simulink model "Learning_Rate"  (R2021b)
settings: Solver=FixedStepAuto  StartTime=0.0  StopTime=1190  FixedStep=0.01  RelTol=1e-3
libraries: drivingcycle_lib x3
settings Model: Creator=Alireza  LastModifiedBy=Alireza

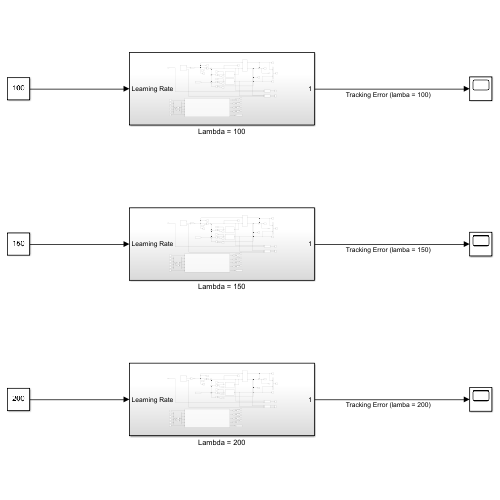
[thumbnail: Simulink's stored preview of the top-level diagram]
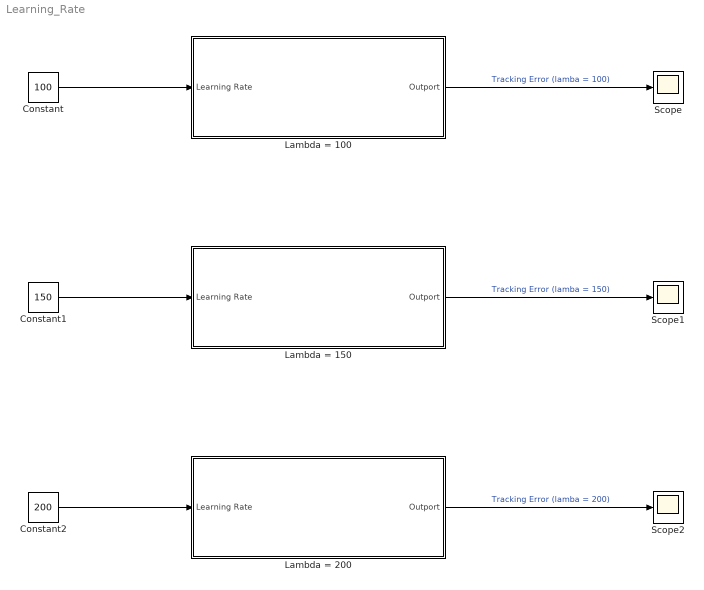
== system Learning_Rate ==
  Constant : Constant  Value=100
  Constant1 : Constant  Value=150
  Constant2 : Constant  Value=200
  Lambda = 100 : Subsystem
  Lambda = 150 : Subsystem
  Lambda = 200 : Subsystem
  Scope : Scope
  Scope1 : Scope
  Scope2 : Scope
  wires:
  Constant/1 -> Lambda = 100/1(Learning Rate)
  Constant1/1 -> Lambda = 150/1(Learning Rate)
  Constant2/1 -> Lambda = 200/1(Learning Rate)
  Lambda = 100/1(Outport) -> Scope/1  "Tracking Error (lamba = 100)"
  Lambda = 150/1(Outport) -> Scope1/1  "Tracking Error (lamba = 150)"
  Lambda = 200/1(Outport) -> Scope2/1  "Tracking Error (lamba = 200)"

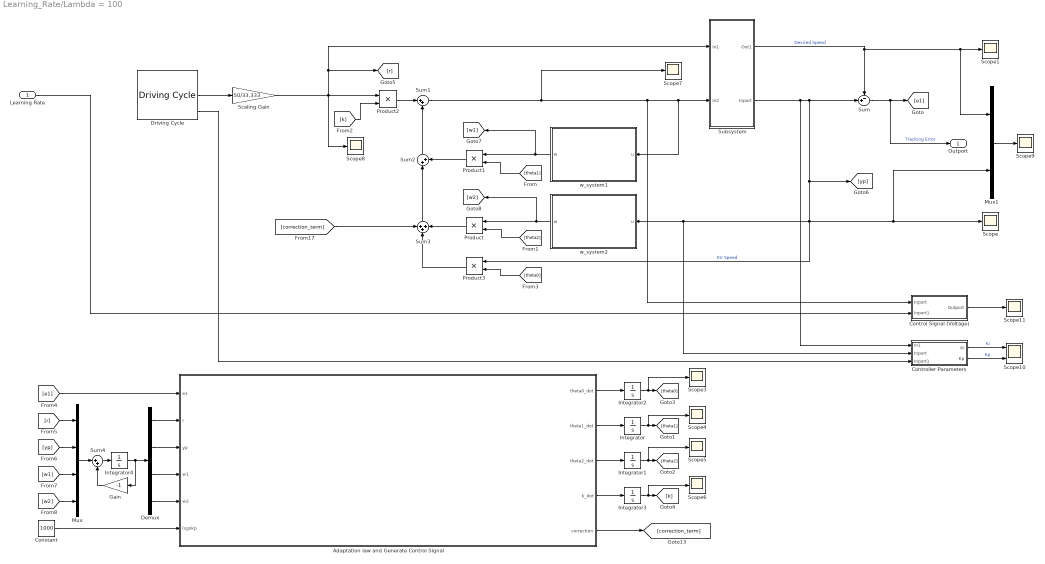
== system Learning_Rate/Lambda = 100 ==
  Learning Rate : Inport
  Adaptation law and Generate Control Signal : MATLAB Function  TreatAsAtomicUnit=on
  Constant : Constant  Value=1000
  Control Signal (Voltage) : Subsystem
  Controller Parameters : Subsystem
  Demux : Demux
  Driving Cycle : drivingcycle_lib/Driving Cycle  CycleName=NEDC  CycleRepeatsForever=off
      settings: SourceProductName=Driving Cycle Blockset
  Gain : Gain  Gain=-1
  Integrator{,1..4} (5 alike) : Integrator
  Mux : Mux
  Mux1 : Mux  Inputs=2
  Product{,1..3} (4 alike) : Product
  Scaling Gain : Gain  Gain=50/33.333
  Scope{,1,3..9,11} (10 alike) : Scope
  Scope10 : Scope  NumInputPorts=2
  Subsystem : Subsystem
  Sum : Sum  Inputs=-+|
  Sum1 : Sum  Inputs=|++
  Sum2 : Sum  Inputs=|++
  Sum3 : Sum  Inputs=+++
  Sum4 : Sum  Inputs=|++
  w_system1 : Subsystem  mask{lambda=-1, l=1}
      mask DialogControl lambda_name Prompt: Lambda:
      mask DialogControl l_name Prompt: L:
  w_system2 : Subsystem  mask{lambda=-1, l=1}
      mask DialogControl lambda_name Prompt: Lambda:
      mask DialogControl l_name Prompt: L:
  Outport : Outport
  wires:
  Subsystem/2(Inport) -> Controller Parameters/1(In1), Controller Parameters/2(Inport), w_system2/1(u), Product3/1, Mux1/2, Scope/1, [yp], Sum/2  "EV Speed"
  [w2] -> Mux/4
  Controller Parameters/2(Kp) -> Scope10/2  "Kp"
  Mux/1 -> Sum4/1
  Control Signal (Voltage)/1(Outport) -> Scope11/1
  Driving Cycle/2 -> Scaling Gain/1
  [e1] -> Adaptation law and Generate Control Signal/1(e1)
  Adaptation law and Generate Control Signal/1(theta0_dot) -> Integrator2/1
  Product/1 -> Sum3/3
  Integrator4/1 -> Gain/1, Demux/1
  Driving Cycle/3 -> Controller Parameters/3(Inport1)
  Controller Parameters/1(Ki) -> Scope10/1  "Ki"
  [correction_term] -> Sum3/1
  Gain/1 -> Sum4/2
  Sum1/1 -> Scope7/1, Control Signal (Voltage)/1(Inport), w_system1/1(u), Subsystem/2(In2)
  Adaptation law and Generate Control Signal/3(theta2_dot) -> Integrator1/1
  Product2/1 -> Sum1/1
  Integrator/1 -> Scope4/1, [theta1]
  w_system1/1(w) -> [w1], Product1/1
  Demux/3 -> Adaptation law and Generate Control Signal/4(w1)
  [r] -> Mux/1
  Product3/1 -> Sum3/2
  Demux/1 -> Adaptation law and Generate Control Signal/2(r)
  w_system2/1(w) -> [w2], Product/1
  Sum4/1 -> Integrator4/1
  Sum/1 -> Outport/1, [e1]  "Tracking Error"
  Subsystem/1(Out1) -> Sum/1, Mux1/1, Scope1/1  "Desired Speed"
  [theta0] -> Product3/2
  Sum2/1 -> Sum1/2
  Adaptation law and Generate Control Signal/4(k_dot) -> Integrator3/1
  [yp] -> Mux/2
  Demux/2 -> Adaptation law and Generate Control Signal/3(yp)
  Sum3/1 -> Sum2/1
  [k] -> Product2/2
  Adaptation law and Generate Control Signal/2(theta1_dot) -> Integrator/1
  Integrator3/1 -> Scope6/1, [k]
  [theta2] -> Product/2
  Mux1/1 -> Scope9/1
  Product1/1 -> Sum2/2
  [w1] -> Mux/3
  [theta1] -> Product1/2
  Adaptation law and Generate Control Signal/5(correction) -> [correction_term]
  Demux/4 -> Adaptation law and Generate Control Signal/5(w2)
  Integrator1/1 -> [theta2], Scope5/1
  Scaling Gain/1 -> Scope8/1, Subsystem/1(In1), [r], Product2/1
  Integrator2/1 -> [theta0], Scope3/1
  Constant/1 -> Adaptation law and Generate Control Signal/6(lsgnkp)
  Learning Rate/1 -> Control Signal (Voltage)/2(Inport1)

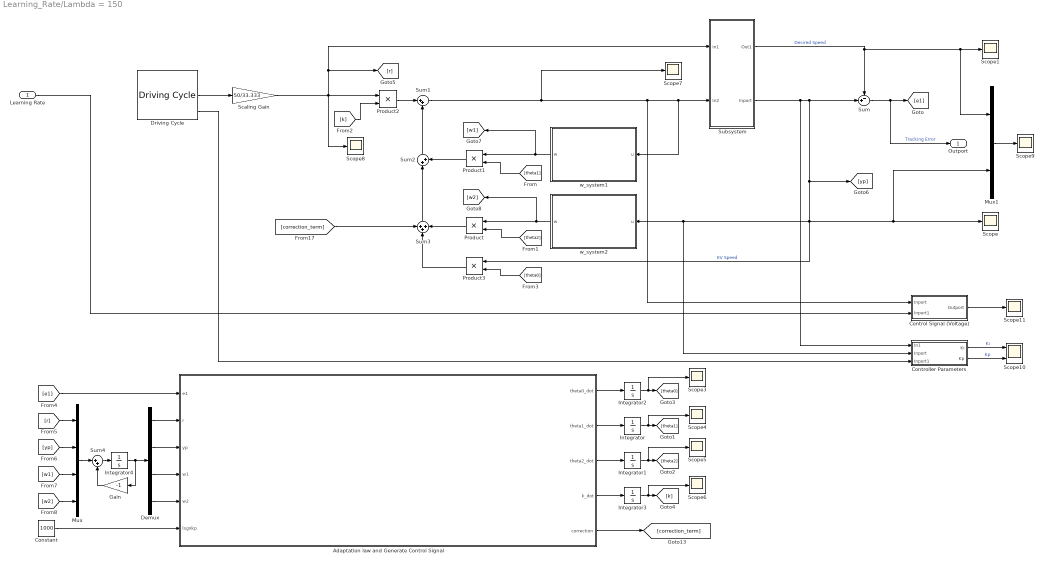
== system Learning_Rate/Lambda = 150 ==
  Learning Rate : Inport
  Adaptation law and Generate Control Signal : MATLAB Function  TreatAsAtomicUnit=on
  Constant : Constant  Value=1000
  Control Signal (Voltage) : Subsystem
  Controller Parameters : Subsystem
  Demux : Demux
  Driving Cycle : drivingcycle_lib/Driving Cycle  CycleName=NEDC  CycleRepeatsForever=off
      settings: SourceProductName=Driving Cycle Blockset
  Gain : Gain  Gain=-1
  Integrator{,1..4} (5 alike) : Integrator
  Mux : Mux
  Mux1 : Mux  Inputs=2
  Product{,1..3} (4 alike) : Product
  Scaling Gain : Gain  Gain=50/33.333
  Scope{,1,3..9,11} (10 alike) : Scope
  Scope10 : Scope  NumInputPorts=2
  Subsystem : Subsystem
  Sum : Sum  Inputs=-+|
  Sum1 : Sum  Inputs=|++
  Sum2 : Sum  Inputs=|++
  Sum3 : Sum  Inputs=+++
  Sum4 : Sum  Inputs=|++
  w_system1 : Subsystem  mask{lambda=-1, l=1}
      mask DialogControl lambda_name Prompt: Lambda:
      mask DialogControl l_name Prompt: L:
  w_system2 : Subsystem  mask{lambda=-1, l=1}
      mask DialogControl lambda_name Prompt: Lambda:
      mask DialogControl l_name Prompt: L:
  Outport : Outport
  wires:
  Subsystem/2(Inport) -> Controller Parameters/1(In1), Controller Parameters/2(Inport), w_system2/1(u), Product3/1, Mux1/2, Scope/1, [yp], Sum/2  "EV Speed"
  [w2] -> Mux/4
  Controller Parameters/2(Kp) -> Scope10/2  "Kp"
  Mux/1 -> Sum4/1
  Control Signal (Voltage)/1(Outport) -> Scope11/1
  Driving Cycle/2 -> Scaling Gain/1
  [e1] -> Adaptation law and Generate Control Signal/1(e1)
  Adaptation law and Generate Control Signal/1(theta0_dot) -> Integrator2/1
  Product/1 -> Sum3/3
  Integrator4/1 -> Gain/1, Demux/1
  Driving Cycle/3 -> Controller Parameters/3(Inport1)
  Controller Parameters/1(Ki) -> Scope10/1  "Ki"
  [correction_term] -> Sum3/1
  Gain/1 -> Sum4/2
  Sum1/1 -> Scope7/1, Control Signal (Voltage)/1(Inport), w_system1/1(u), Subsystem/2(In2)
  Adaptation law and Generate Control Signal/3(theta2_dot) -> Integrator1/1
  Product2/1 -> Sum1/1
  Integrator/1 -> Scope4/1, [theta1]
  w_system1/1(w) -> [w1], Product1/1
  Demux/3 -> Adaptation law and Generate Control Signal/4(w1)
  [r] -> Mux/1
  Product3/1 -> Sum3/2
  Demux/1 -> Adaptation law and Generate Control Signal/2(r)
  w_system2/1(w) -> [w2], Product/1
  Sum4/1 -> Integrator4/1
  Sum/1 -> Outport/1, [e1]  "Tracking Error"
  Subsystem/1(Out1) -> Sum/1, Mux1/1, Scope1/1  "Desired Speed"
  [theta0] -> Product3/2
  Sum2/1 -> Sum1/2
  Adaptation law and Generate Control Signal/4(k_dot) -> Integrator3/1
  [yp] -> Mux/2
  Demux/2 -> Adaptation law and Generate Control Signal/3(yp)
  Sum3/1 -> Sum2/1
  [k] -> Product2/2
  Adaptation law and Generate Control Signal/2(theta1_dot) -> Integrator/1
  Integrator3/1 -> Scope6/1, [k]
  [theta2] -> Product/2
  Mux1/1 -> Scope9/1
  Product1/1 -> Sum2/2
  [w1] -> Mux/3
  [theta1] -> Product1/2
  Adaptation law and Generate Control Signal/5(correction) -> [correction_term]
  Demux/4 -> Adaptation law and Generate Control Signal/5(w2)
  Integrator1/1 -> [theta2], Scope5/1
  Scaling Gain/1 -> Scope8/1, Subsystem/1(In1), [r], Product2/1
  Integrator2/1 -> [theta0], Scope3/1
  Constant/1 -> Adaptation law and Generate Control Signal/6(lsgnkp)
  Learning Rate/1 -> Control Signal (Voltage)/2(Inport1)

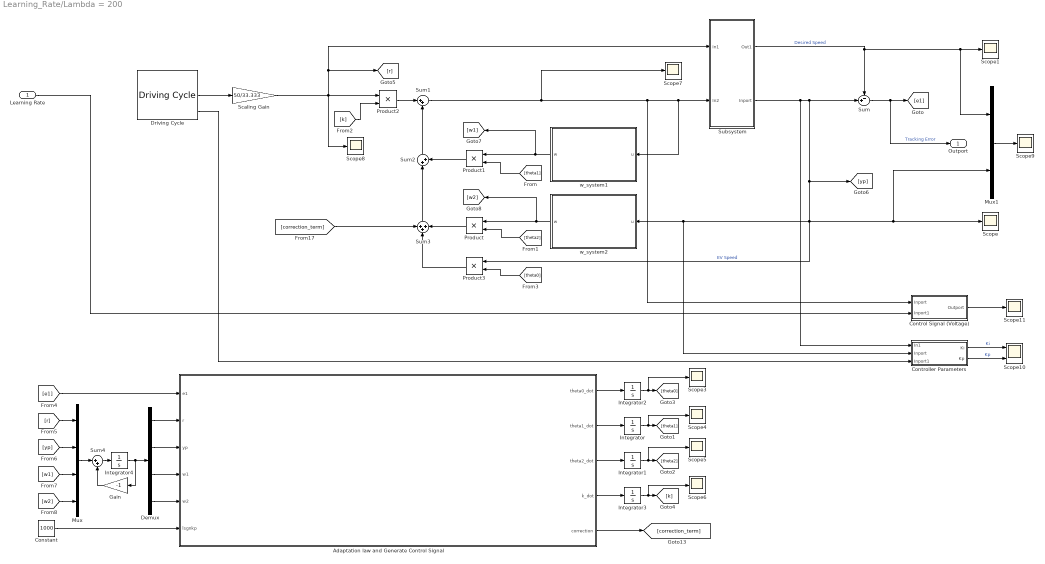
== system Learning_Rate/Lambda = 200 ==
  Learning Rate : Inport
  Adaptation law and Generate Control Signal : MATLAB Function  TreatAsAtomicUnit=on
  Constant : Constant  Value=1000
  Control Signal (Voltage) : Subsystem
  Controller Parameters : Subsystem
  Demux : Demux
  Driving Cycle : drivingcycle_lib/Driving Cycle  CycleName=NEDC  CycleRepeatsForever=off
      settings: SourceProductName=Driving Cycle Blockset
  Gain : Gain  Gain=-1
  Integrator{,1..4} (5 alike) : Integrator
  Mux : Mux
  Mux1 : Mux  Inputs=2
  Product{,1..3} (4 alike) : Product
  Scaling Gain : Gain  Gain=50/33.333
  Scope{,1,3..9,11} (10 alike) : Scope
  Scope10 : Scope  NumInputPorts=2
  Subsystem : Subsystem
  Sum : Sum  Inputs=-+|
  Sum1 : Sum  Inputs=|++
  Sum2 : Sum  Inputs=|++
  Sum3 : Sum  Inputs=+++
  Sum4 : Sum  Inputs=|++
  w_system1 : Subsystem  mask{lambda=-1, l=1}
      mask DialogControl lambda_name Prompt: Lambda:
      mask DialogControl l_name Prompt: L:
  w_system2 : Subsystem  mask{lambda=-1, l=1}
      mask DialogControl lambda_name Prompt: Lambda:
      mask DialogControl l_name Prompt: L:
  Outport : Outport
  wires:
  Subsystem/2(Inport) -> Controller Parameters/1(In1), Controller Parameters/2(Inport), w_system2/1(u), Product3/1, Mux1/2, Scope/1, [yp], Sum/2  "EV Speed"
  [w2] -> Mux/4
  Controller Parameters/2(Kp) -> Scope10/2  "Kp"
  Mux/1 -> Sum4/1
  Control Signal (Voltage)/1(Outport) -> Scope11/1
  Driving Cycle/2 -> Scaling Gain/1
  [e1] -> Adaptation law and Generate Control Signal/1(e1)
  Adaptation law and Generate Control Signal/1(theta0_dot) -> Integrator2/1
  Product/1 -> Sum3/3
  Integrator4/1 -> Gain/1, Demux/1
  Driving Cycle/3 -> Controller Parameters/3(Inport1)
  Controller Parameters/1(Ki) -> Scope10/1  "Ki"
  [correction_term] -> Sum3/1
  Gain/1 -> Sum4/2
  Sum1/1 -> Scope7/1, Control Signal (Voltage)/1(Inport), w_system1/1(u), Subsystem/2(In2)
  Adaptation law and Generate Control Signal/3(theta2_dot) -> Integrator1/1
  Product2/1 -> Sum1/1
  Integrator/1 -> Scope4/1, [theta1]
  w_system1/1(w) -> [w1], Product1/1
  Demux/3 -> Adaptation law and Generate Control Signal/4(w1)
  [r] -> Mux/1
  Product3/1 -> Sum3/2
  Demux/1 -> Adaptation law and Generate Control Signal/2(r)
  w_system2/1(w) -> [w2], Product/1
  Sum4/1 -> Integrator4/1
  Sum/1 -> Outport/1, [e1]  "Tracking Error"
  Subsystem/1(Out1) -> Sum/1, Mux1/1, Scope1/1  "Desired Speed"
  [theta0] -> Product3/2
  Sum2/1 -> Sum1/2
  Adaptation law and Generate Control Signal/4(k_dot) -> Integrator3/1
  [yp] -> Mux/2
  Demux/2 -> Adaptation law and Generate Control Signal/3(yp)
  Sum3/1 -> Sum2/1
  [k] -> Product2/2
  Adaptation law and Generate Control Signal/2(theta1_dot) -> Integrator/1
  Integrator3/1 -> Scope6/1, [k]
  [theta2] -> Product/2
  Mux1/1 -> Scope9/1
  Product1/1 -> Sum2/2
  [w1] -> Mux/3
  [theta1] -> Product1/2
  Adaptation law and Generate Control Signal/5(correction) -> [correction_term]
  Demux/4 -> Adaptation law and Generate Control Signal/5(w2)
  Integrator1/1 -> [theta2], Scope5/1
  Scaling Gain/1 -> Scope8/1, Subsystem/1(In1), [r], Product2/1
  Integrator2/1 -> [theta0], Scope3/1
  Constant/1 -> Adaptation law and Generate Control Signal/6(lsgnkp)
  Learning Rate/1 -> Control Signal (Voltage)/2(Inport1)

== system Learning_Rate/Lambda = 100/Control Signal (Voltage) ==
  Inport : Inport
  Inport1 : Inport  Port=2
  Outport : Outport
  wires:
  Inport/1 -> Outport/1

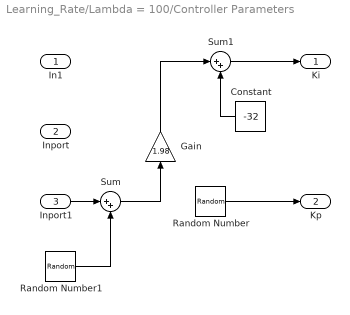
== system Learning_Rate/Lambda = 100/Controller Parameters ==
  In1 : Inport
  Inport : Inport  Port=2
  Inport1 : Inport  Port=3
  Constant : Constant  Value=-32
  Gain : Gain  Gain=1.98
  Random Number : RandomNumber  Mean=165  Variance=0.05  SampleTime=0.1
  Random Number1 : RandomNumber  Mean=67  Variance=0.001  SampleTime=0.1
  Sum : Sum  Inputs=|++
  Sum1 : Sum  Inputs=|++
  Ki : Outport
  Kp : Outport  Port=2
  wires:
  Random Number/1 -> Kp/1
  Inport1/1 -> Sum/1
  Random Number1/1 -> Sum/2
  Sum/1 -> Gain/1
  Gain/1 -> Sum1/1
  Constant/1 -> Sum1/2
  Sum1/1 -> Ki/1

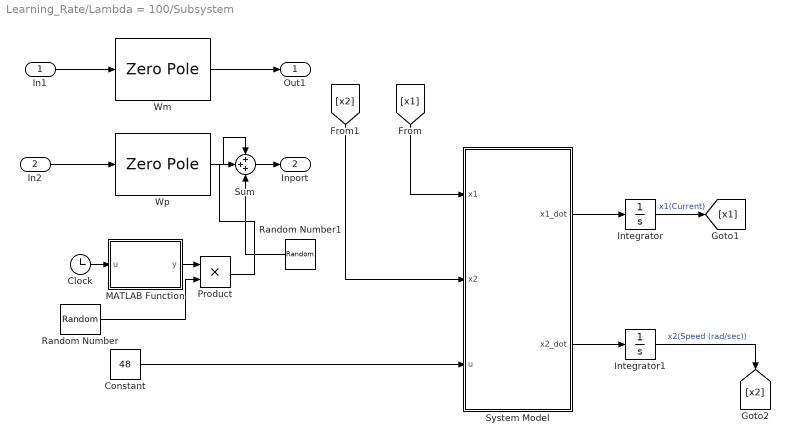
== system Learning_Rate/Lambda = 100/Subsystem ==
  In1 : Inport
  In2 : Inport  Port=2
  Clock : Clock
  Constant : Constant  Value=48
  Integrator : Integrator  InitialCondition=5
  Integrator1 : Integrator
  MATLAB Function : MATLAB Function  TreatAsAtomicUnit=on
  Product : Product
  Random Number : RandomNumber  Variance=0.007  SampleTime=0.1
  Random Number1 : RandomNumber  Variance=0.0005  SampleTime=0.1
  Sum : Sum  Inputs=+++
  System Model : MATLAB Function  TreatAsAtomicUnit=on
  Wm : ZeroPole  Zeros=[]  Poles=[-1 -1]
  Wp : ZeroPole  Zeros=[]
  Out1 : Outport
  Inport : Outport  Port=2
  wires:
  In2/1 -> Wp/1
  In1/1 -> Wm/1
  Wm/1 -> Out1/1
  Constant/1 -> System Model/3(u)
  Integrator/1 -> [x1]  "x1(Current)"
  [x1] -> System Model/1(x1)
  Integrator1/1 -> [x2]  "x2(Speed (rad/sec))"
  System Model/2(x2_dot) -> Integrator1/1
  System Model/1(x1_dot) -> Integrator/1
  [x2] -> System Model/2(x2)
  Wp/1 -> Sum/1
  Sum/1 -> Inport/1
  Clock/1 -> MATLAB Function/1(u)
  MATLAB Function/1(y) -> Product/1
  Random Number/1 -> Product/2
  Product/1 -> Sum/2
  Random Number1/1 -> Sum/3

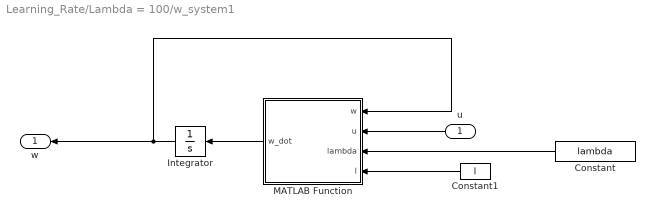
== system Learning_Rate/Lambda = 100/w_system1 ==
  u : Inport
  Constant : Constant  Value=lambda
  Constant1 : Constant  Value=l
  Integrator : Integrator  InitialCondition=zeros(size(l,1),1)
  MATLAB Function : MATLAB Function  TreatAsAtomicUnit=on
  w : Outport  VectorParamsAs1DForOutWhenUnconnected=off
  wires:
  Constant1/1 -> MATLAB Function/4(l)
  Constant/1 -> MATLAB Function/3(lambda)
  u/1 -> MATLAB Function/2(u)
  MATLAB Function/1(w_dot) -> Integrator/1
  Integrator/1 -> MATLAB Function/1(w), w/1

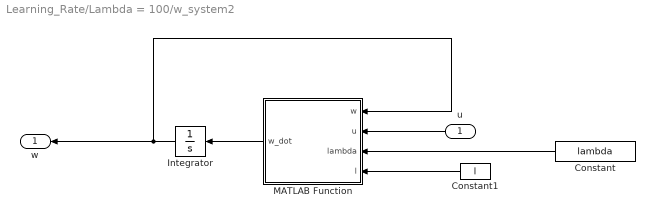
== system Learning_Rate/Lambda = 100/w_system2 ==
  u : Inport
  Constant : Constant  Value=lambda
  Constant1 : Constant  Value=l
  Integrator : Integrator  InitialCondition=zeros(size(l,1),1)
  MATLAB Function : MATLAB Function  TreatAsAtomicUnit=on
  w : Outport  VectorParamsAs1DForOutWhenUnconnected=off
  wires:
  Integrator/1 -> w/1, MATLAB Function/1(w)
  MATLAB Function/1(w_dot) -> Integrator/1
  u/1 -> MATLAB Function/2(u)
  Constant/1 -> MATLAB Function/3(lambda)
  Constant1/1 -> MATLAB Function/4(l)

== system Learning_Rate/Lambda = 150/Control Signal (Voltage) ==
  Inport : Inport
  Inport1 : Inport  Port=2
  Outport : Outport
  wires:
  Inport/1 -> Outport/1

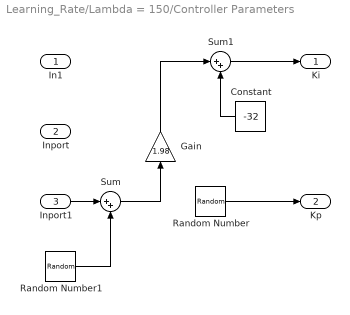
== system Learning_Rate/Lambda = 150/Controller Parameters ==
  In1 : Inport
  Inport : Inport  Port=2
  Inport1 : Inport  Port=3
  Constant : Constant  Value=-32
  Gain : Gain  Gain=1.98
  Random Number : RandomNumber  Mean=165  Variance=0.05  SampleTime=0.1
  Random Number1 : RandomNumber  Mean=67  Variance=0.001  SampleTime=0.1
  Sum : Sum  Inputs=|++
  Sum1 : Sum  Inputs=|++
  Ki : Outport
  Kp : Outport  Port=2
  wires:
  Random Number/1 -> Kp/1
  Inport1/1 -> Sum/1
  Random Number1/1 -> Sum/2
  Sum/1 -> Gain/1
  Gain/1 -> Sum1/1
  Constant/1 -> Sum1/2
  Sum1/1 -> Ki/1

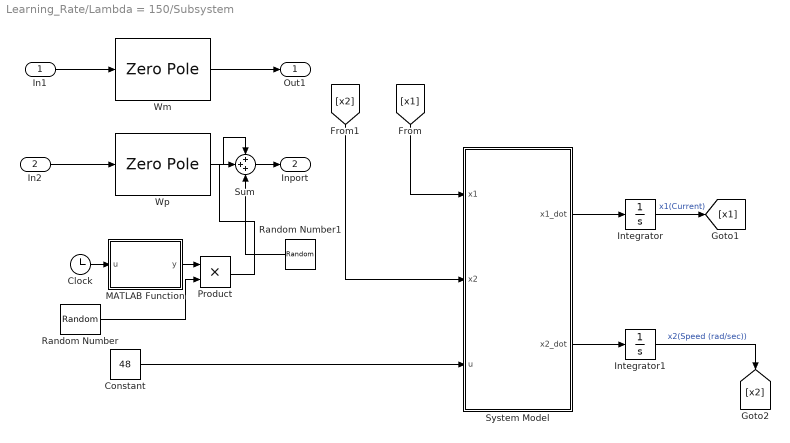
== system Learning_Rate/Lambda = 150/Subsystem ==
  In1 : Inport
  In2 : Inport  Port=2
  Clock : Clock
  Constant : Constant  Value=48
  Integrator : Integrator  InitialCondition=5
  Integrator1 : Integrator
  MATLAB Function : MATLAB Function  TreatAsAtomicUnit=on
  Product : Product
  Random Number : RandomNumber  Variance=0.003  SampleTime=0.1
  Random Number1 : RandomNumber  Variance=0.0003  SampleTime=0.1
  Sum : Sum  Inputs=+++
  System Model : MATLAB Function  TreatAsAtomicUnit=on
  Wm : ZeroPole  Zeros=[]  Poles=[-1 -1]
  Wp : ZeroPole  Zeros=[]
  Out1 : Outport
  Inport : Outport  Port=2
  wires:
  In2/1 -> Wp/1
  In1/1 -> Wm/1
  Wm/1 -> Out1/1
  Constant/1 -> System Model/3(u)
  Integrator/1 -> [x1]  "x1(Current)"
  [x1] -> System Model/1(x1)
  Integrator1/1 -> [x2]  "x2(Speed (rad/sec))"
  System Model/2(x2_dot) -> Integrator1/1
  System Model/1(x1_dot) -> Integrator/1
  [x2] -> System Model/2(x2)
  Wp/1 -> Sum/1
  Sum/1 -> Inport/1
  Clock/1 -> MATLAB Function/1(u)
  MATLAB Function/1(y) -> Product/1
  Random Number/1 -> Product/2
  Product/1 -> Sum/2
  Random Number1/1 -> Sum/3

== system Learning_Rate/Lambda = 150/w_system1 ==
  u : Inport
  Constant : Constant  Value=lambda
  Constant1 : Constant  Value=l
  Integrator : Integrator  InitialCondition=zeros(size(l,1),1)
  MATLAB Function : MATLAB Function  TreatAsAtomicUnit=on
  w : Outport  VectorParamsAs1DForOutWhenUnconnected=off
  wires:
  Constant1/1 -> MATLAB Function/4(l)
  Constant/1 -> MATLAB Function/3(lambda)
  u/1 -> MATLAB Function/2(u)
  MATLAB Function/1(w_dot) -> Integrator/1
  Integrator/1 -> MATLAB Function/1(w), w/1

== system Learning_Rate/Lambda = 150/w_system2 ==
  u : Inport
  Constant : Constant  Value=lambda
  Constant1 : Constant  Value=l
  Integrator : Integrator  InitialCondition=zeros(size(l,1),1)
  MATLAB Function : MATLAB Function  TreatAsAtomicUnit=on
  w : Outport  VectorParamsAs1DForOutWhenUnconnected=off
  wires:
  Integrator/1 -> w/1, MATLAB Function/1(w)
  MATLAB Function/1(w_dot) -> Integrator/1
  u/1 -> MATLAB Function/2(u)
  Constant/1 -> MATLAB Function/3(lambda)
  Constant1/1 -> MATLAB Function/4(l)

== system Learning_Rate/Lambda = 200/Control Signal (Voltage) ==
  Inport : Inport
  Inport1 : Inport  Port=2
  Outport : Outport
  wires:
  Inport/1 -> Outport/1

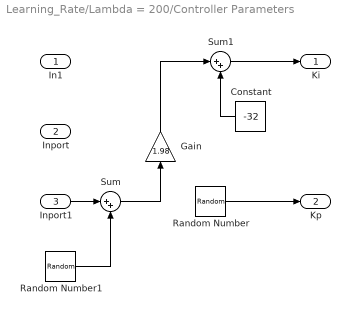
== system Learning_Rate/Lambda = 200/Controller Parameters ==
  In1 : Inport
  Inport : Inport  Port=2
  Inport1 : Inport  Port=3
  Constant : Constant  Value=-32
  Gain : Gain  Gain=1.98
  Random Number : RandomNumber  Mean=165  Variance=0.05  SampleTime=0.1
  Random Number1 : RandomNumber  Mean=67  Variance=0.001  SampleTime=0.1
  Sum : Sum  Inputs=|++
  Sum1 : Sum  Inputs=|++
  Ki : Outport
  Kp : Outport  Port=2
  wires:
  Random Number/1 -> Kp/1
  Inport1/1 -> Sum/1
  Random Number1/1 -> Sum/2
  Sum/1 -> Gain/1
  Gain/1 -> Sum1/1
  Constant/1 -> Sum1/2
  Sum1/1 -> Ki/1

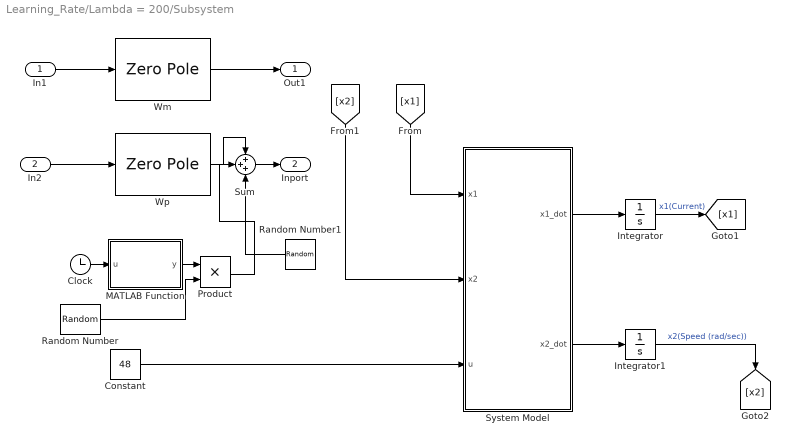
== system Learning_Rate/Lambda = 200/Subsystem ==
  In1 : Inport
  In2 : Inport  Port=2
  Clock : Clock
  Constant : Constant  Value=48
  Integrator : Integrator  InitialCondition=5
  Integrator1 : Integrator
  MATLAB Function : MATLAB Function  TreatAsAtomicUnit=on
  Product : Product
  Random Number : RandomNumber  Variance=0.002  SampleTime=0.1
  Random Number1 : RandomNumber  Variance=0.0005  SampleTime=0.1
  Sum : Sum  Inputs=+++
  System Model : MATLAB Function  TreatAsAtomicUnit=on
  Wm : ZeroPole  Zeros=[]  Poles=[-1 -1]
  Wp : ZeroPole  Zeros=[]
  Out1 : Outport
  Inport : Outport  Port=2
  wires:
  In2/1 -> Wp/1
  In1/1 -> Wm/1
  Wm/1 -> Out1/1
  Constant/1 -> System Model/3(u)
  Integrator/1 -> [x1]  "x1(Current)"
  [x1] -> System Model/1(x1)
  Integrator1/1 -> [x2]  "x2(Speed (rad/sec))"
  System Model/2(x2_dot) -> Integrator1/1
  System Model/1(x1_dot) -> Integrator/1
  [x2] -> System Model/2(x2)
  Wp/1 -> Sum/1
  Sum/1 -> Inport/1
  Clock/1 -> MATLAB Function/1(u)
  MATLAB Function/1(y) -> Product/1
  Random Number/1 -> Product/2
  Product/1 -> Sum/2
  Random Number1/1 -> Sum/3

== system Learning_Rate/Lambda = 200/w_system1 ==
  u : Inport
  Constant : Constant  Value=lambda
  Constant1 : Constant  Value=l
  Integrator : Integrator  InitialCondition=zeros(size(l,1),1)
  MATLAB Function : MATLAB Function  TreatAsAtomicUnit=on
  w : Outport  VectorParamsAs1DForOutWhenUnconnected=off
  wires:
  Constant1/1 -> MATLAB Function/4(l)
  Constant/1 -> MATLAB Function/3(lambda)
  u/1 -> MATLAB Function/2(u)
  MATLAB Function/1(w_dot) -> Integrator/1
  Integrator/1 -> MATLAB Function/1(w), w/1

== system Learning_Rate/Lambda = 200/w_system2 ==
  u : Inport
  Constant : Constant  Value=lambda
  Constant1 : Constant  Value=l
  Integrator : Integrator  InitialCondition=zeros(size(l,1),1)
  MATLAB Function : MATLAB Function  TreatAsAtomicUnit=on
  w : Outport  VectorParamsAs1DForOutWhenUnconnected=off
  wires:
  Integrator/1 -> w/1, MATLAB Function/1(w)
  MATLAB Function/1(w_dot) -> Integrator/1
  u/1 -> MATLAB Function/2(u)
  Constant/1 -> MATLAB Function/3(lambda)
  Constant1/1 -> MATLAB Function/4(l)

== matlab function Learning_Rate/Lambda = 150/w_system1/MATLAB Function ==
  data: w input; u input; w_dot output; lambda input; l input
function w_dot = fcn(w , u , lambda , l)

w_dot = lambda*w + l*u; 
end

== matlab function Learning_Rate/Lambda = 150/w_system2/MATLAB Function ==
  data: w input; u input; w_dot output; lambda input; l input
function w_dot = fcn(w , u , lambda , l)

w_dot = lambda*w + l*u; 
end

== matlab function Learning_Rate/Lambda = 200/Adaptation law and Generate Control Signal ==
  data: e1 input; theta0_dot output; r input; yp input; w1 input; w2 input; theta1_dot output; theta2_dot output; k_dot output; lsgnkp input; correction output
function [theta0_dot , theta1_dot , theta2_dot , k_dot , correction] = fcn(e1 ,r , yp , w1 , w2 , lsgnkp)

theta0_dot = -lsgnkp*e1*yp;
theta1_dot = -lsgnkp*e1*w1;
theta2_dot = -lsgnkp*e1*w2;
k_dot = -lsgnkp*e1*r;

W = [r yp w1 w2].';
THETA_T = [k_dot theta0_dot theta1_dot theta2_dot];

correction = THETA_T*W;
end

== matlab function Learning_Rate/Lambda = 200/Subsystem/MATLAB Function ==
  data: u input; y output
function y = fcn(u)

y = exp(-0.3*u);

== matlab function Learning_Rate/Lambda = 200/Subsystem/System Model ==
  data: x1 input; x1_dot output; x2 input; u input; x2_dot output
function [x1_dot, x2_dot]= fcn(x1, x2, u)
Ra_plus_Rf = 0.12;      % Armature and Field Resistance
La_plus_Lf = 6.008e-3;  % Armature and Field Inductance
r = 0.25;               % Wheel Radious
J = 0.05;               % Inertai of the Motor
L_af = 1.766e-3;        % Mutual Inductance
I = 78;                 % Maximum Current
omega_norm = 2800;      % Nominal omega
m = 800;                % Total mass (kg)
A = 1.8;                % Frontal Area of the Vegicle
ro = 1.25;              % Air density
Cd = 0.3;               % Drag Coefficient
phi = 0;                % Hill climbing Angle
mu_rr = 0.015;          % Rolling Resistance Coefficient
G = 11;                 % Gearbox Ratio
B = 0.0002;             % Viscous Coefficient
g = 9.8;                % Gravity Constant 
V = 48;                 % Input Voltage  0 ~ 48 volt

x1_dot = (1/La_plus_Lf) * (-(Ra_plus_Rf) * x1 - L_af * x1 * x2) + (1/La_plus_Lf) * u;
x2_dot = (1 / (J + m * (r/G)^2)) * (L_af * x1^2 -B * x2 - (r/G) * (mu_rr * m * g + 0.5 * ro * A * Cd * (r/G)^2 * x2^2 + m*g*sin(phi)));


end

== matlab function Learning_Rate/Lambda = 200/w_system1/MATLAB Function ==
  data: w input; u input; w_dot output; lambda input; l input
function w_dot = fcn(w , u , lambda , l)

w_dot = lambda*w + l*u; 
end

== matlab function Learning_Rate/Lambda = 100/w_system1/MATLAB Function ==
  data: w input; u input; w_dot output; lambda input; l input
function w_dot = fcn(w , u , lambda , l)

w_dot = lambda*w + l*u; 
end

== matlab function Learning_Rate/Lambda = 200/w_system2/MATLAB Function ==
  data: w input; u input; w_dot output; lambda input; l input
function w_dot = fcn(w , u , lambda , l)

w_dot = lambda*w + l*u; 
end

== matlab function Learning_Rate/Lambda = 100/w_system2/MATLAB Function ==
  data: w input; u input; w_dot output; lambda input; l input
function w_dot = fcn(w , u , lambda , l)

w_dot = lambda*w + l*u; 
end

== matlab function Learning_Rate/Lambda = 100/Adaptation law and Generate Control Signal ==
  data: e1 input; theta0_dot output; r input; yp input; w1 input; w2 input; theta1_dot output; theta2_dot output; k_dot output; lsgnkp input; correction output
function [theta0_dot , theta1_dot , theta2_dot , k_dot , correction] = fcn(e1 ,r , yp , w1 , w2 , lsgnkp)

theta0_dot = -lsgnkp*e1*yp;
theta1_dot = -lsgnkp*e1*w1;
theta2_dot = -lsgnkp*e1*w2;
k_dot = -lsgnkp*e1*r;

W = [r yp w1 w2].';
THETA_T = [k_dot theta0_dot theta1_dot theta2_dot];

correction = THETA_T*W;
end

== matlab function Learning_Rate/Lambda = 100/Subsystem/System Model ==
  data: x1 input; x1_dot output; x2 input; u input; x2_dot output
function [x1_dot, x2_dot]= fcn(x1, x2, u)
Ra_plus_Rf = 0.12;      % Armature and Field Resistance
La_plus_Lf = 6.008e-3;  % Armature and Field Inductance
r = 0.25;               % Wheel Radious
J = 0.05;               % Inertai of the Motor
L_af = 1.766e-3;        % Mutual Inductance
I = 78;                 % Maximum Current
omega_norm = 2800;      % Nominal omega
m = 800;                % Total mass (kg)
A = 1.8;                % Frontal Area of the Vegicle
ro = 1.25;              % Air density
Cd = 0.3;               % Drag Coefficient
phi = 0;                % Hill climbing Angle
mu_rr = 0.015;          % Rolling Resistance Coefficient
G = 11;                 % Gearbox Ratio
B = 0.0002;             % Viscous Coefficient
g = 9.8;                % Gravity Constant 
V = 48;                 % Input Voltage  0 ~ 48 volt

x1_dot = (1/La_plus_Lf) * (-(Ra_plus_Rf) * x1 - L_af * x1 * x2) + (1/La_plus_Lf) * u;
x2_dot = (1 / (J + m * (r/G)^2)) * (L_af * x1^2 -B * x2 - (r/G) * (mu_rr * m * g + 0.5 * ro * A * Cd * (r/G)^2 * x2^2 + m*g*sin(phi)));


end

== matlab function Learning_Rate/Lambda = 100/Subsystem/MATLAB Function ==
  data: u input; y output
function y = fcn(u)

y = exp(-0.3*u);

== matlab function Learning_Rate/Lambda = 150/Adaptation law and Generate Control Signal ==
  data: e1 input; theta0_dot output; r input; yp input; w1 input; w2 input; theta1_dot output; theta2_dot output; k_dot output; lsgnkp input; correction output
function [theta0_dot , theta1_dot , theta2_dot , k_dot , correction] = fcn(e1 ,r , yp , w1 , w2 , lsgnkp)

theta0_dot = -lsgnkp*e1*yp;
theta1_dot = -lsgnkp*e1*w1;
theta2_dot = -lsgnkp*e1*w2;
k_dot = -lsgnkp*e1*r;

W = [r yp w1 w2].';
THETA_T = [k_dot theta0_dot theta1_dot theta2_dot];

correction = THETA_T*W;
end

== matlab function Learning_Rate/Lambda = 150/Subsystem/MATLAB Function ==
  data: u input; y output
function y = fcn(u)

y = exp(-0.3*u);

== matlab function Learning_Rate/Lambda = 150/Subsystem/System Model ==
  data: x1 input; x1_dot output; x2 input; u input; x2_dot output
function [x1_dot, x2_dot]= fcn(x1, x2, u)
Ra_plus_Rf = 0.12;      % Armature and Field Resistance
La_plus_Lf = 6.008e-3;  % Armature and Field Inductance
r = 0.25;               % Wheel Radious
J = 0.05;               % Inertai of the Motor
L_af = 1.766e-3;        % Mutual Inductance
I = 78;                 % Maximum Current
omega_norm = 2800;      % Nominal omega
m = 800;                % Total mass (kg)
A = 1.8;                % Frontal Area of the Vegicle
ro = 1.25;              % Air density
Cd = 0.3;               % Drag Coefficient
phi = 0;                % Hill climbing Angle
mu_rr = 0.015;          % Rolling Resistance Coefficient
G = 11;                 % Gearbox Ratio
B = 0.0002;             % Viscous Coefficient
g = 9.8;                % Gravity Constant 
V = 48;                 % Input Voltage  0 ~ 48 volt

x1_dot = (1/La_plus_Lf) * (-(Ra_plus_Rf) * x1 - L_af * x1 * x2) + (1/La_plus_Lf) * u;
x2_dot = (1 / (J + m * (r/G)^2)) * (L_af * x1^2 -B * x2 - (r/G) * (mu_rr * m * g + 0.5 * ro * A * Cd * (r/G)^2 * x2^2 + m*g*sin(phi)));


end
